simulink model "Frank_mececaneum"  (R2023b)
settings: Solver=VariableStepAuto  StartTime=0.0  StopTime=10.0  RelTol=1e-3
values from neighbouring files (symbols this model uses):
  qn = [0, pi/4, pi, 0, pi/4, 0]    [OMPro.m]    (also in OMPro_v1.m = [0, -pi/4, 0, 0, pi/4, 0]; OManPro.m = rand(1,6); moron9dof.m = [0.1 0.1 pi/4 pi/4 -pi/4 pi/4 0 pi/4 0]; testing2.m = [0 pi/4 pi/4 0 pi/4 0])
undefined symbols (not defined in the file or in its folder): cinertia, nofriction, p560
libraries: roblocks x8
settings Model: Creator=kangwang  LastModifiedBy=kangwang

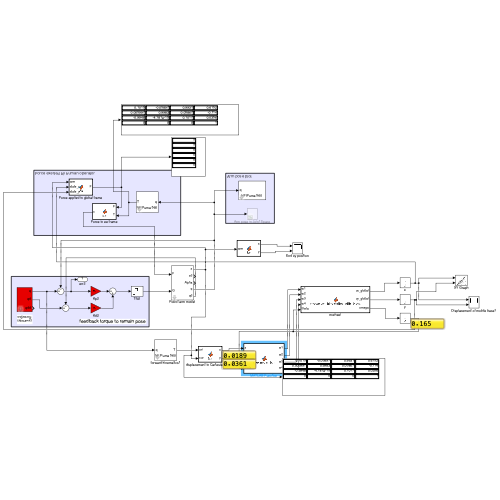
[thumbnail: Simulink's stored preview of the top-level diagram]
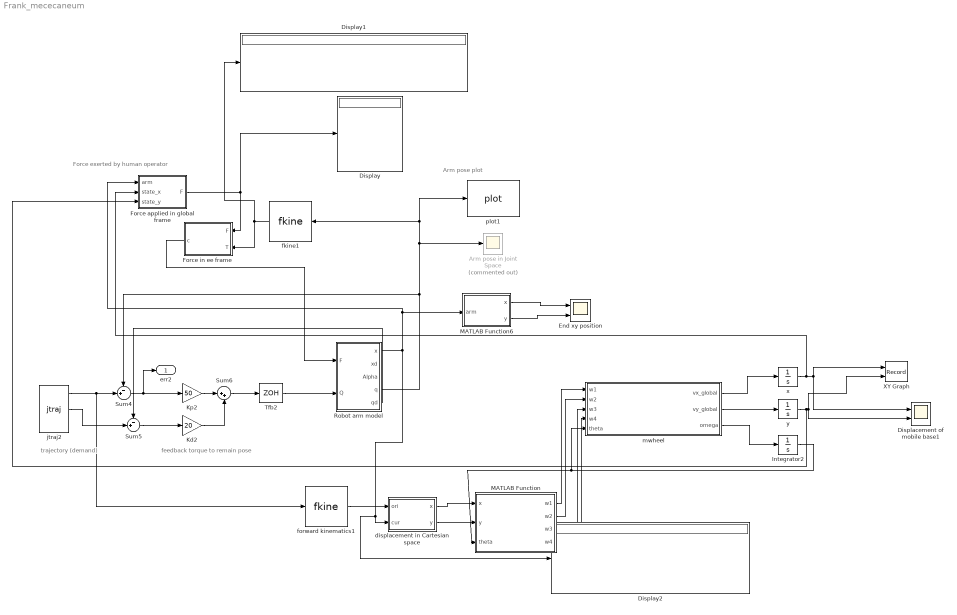
== system Frank_mececaneum ==
  note: feedback torque to remain pose
  note: Force exerted by human operator
  note: trajectory
      | (demand)
  note: Arm pose plot
  Arm pose in Joint Space : Scope  Commented=on
  Displacement of mobile base1 : Scope  NumInputPorts=2
  Display : Display
  Display1 : Display
  Display2 : Display
  End xy position : Scope  NumInputPorts=2
  Force applied in global frame : MATLAB Function  TreatAsAtomicUnit=on
  Force in ee frame : MATLAB Function  TreatAsAtomicUnit=on
  Integrator2 : Integrator
  Kd2 : Gain  Gain=20  SaturateOnIntegerOverflow=on  OutDataTypeStr=Inherit: Same as input  ParamDataTypeStr=Inherit: Same as input
  Kp2 : Gain  Gain=50  SaturateOnIntegerOverflow=on  OutDataTypeStr=Inherit: Same as input  ParamDataTypeStr=Inherit: Same as input
  MATLAB Function : MATLAB Function  TreatAsAtomicUnit=on
  MATLAB Function6 : MATLAB Function  TreatAsAtomicUnit=on
  Robot arm model : Subsystem  mask{robot=nofriction(p560), q0=qn}
      mask prompts: q0 "Initial joint angles"
  Sum4 : Sum  Inputs=-+|  InputSameDT=on  SaturateOnIntegerOverflow=on  OutDataTypeStr=Inherit: Same as first input
  Sum5 : Sum  Inputs=-+|  InputSameDT=on  SaturateOnIntegerOverflow=on  OutDataTypeStr=Inherit: Same as first input
  Sum6 : Sum  Inputs=|++  InputSameDT=on  SaturateOnIntegerOverflow=on  OutDataTypeStr=Inherit: Same as first input
  Tfb2 : ZeroOrderHold  SampleTime=0.002
  XY Graph : Record  FileSettingsInternal="{\"entries\":[{\"content\":{\"excelSettings\":{\"content\":{},\"type\":\"Streamout.ExcelSettings\"}},\"type\":\"Streamout.FileSettingStorage\",\"uuid\":\"\"}],\"packageUris\":[\"http:\\/\\/schema.mathworks.com\\/mf0\\/streamout_blocks\\/R2020a\"],\"version\":\"1.0\"}"  Layout=[1 1]  SignalsInternal="{\"entries\":[{\"content\":{\"signals\":[{\"content\":{\"blockPath\":[],\"dimensions\":[1],\"domain\":\"\",\"lineColor\":\"#a2142f\",\"plots\":[1],\"port\":1,\"sid\":[\"\"],\"signalID\":412,\"signalName\":\"x\"},\"type\":\"RecordBlkView.Signal\",\"uuid\":\"\"},{\"content\":{\"blockPath\":[],\"dimensions\":[1],\"domain\":\"\",\"lineColor\":\"#139fff\",\"plots\":[1],\"port\":2,\"sid\":[\"\"],\"signalID\":416,\"signalName\":\"y\"},\"type\":\"RecordBlkView.Signal\",\"uuid\":\"\"}]},\"type\":\"RecordBlkView.InputSignals\",\"uuid\":\"\"}],\"packageUris\":[\"http:\\/\\/schema.mathworks.com\\/mf0\\/streamout_blocks\\/R2020a\"],\"version\":\"1.0\"}"  VisualizationBindings="{\"xyplotplugin\":{\"info\":[{\"series\":[{\"bindingParametersList\":[{\"parameter\":\"X-Axis\",\"signalID\":412,\"signalName\":\"x\"},{\"parameter\":\"Y-Axis\",\"signalID\":416,\"signalName\":\"y\"}],\"seriesID\":11544}],\"subplotID\":1}]}}"  CompatibilityTag=XY
  displacement in Cartesian space : MATLAB Function  TreatAsAtomicUnit=on
  fkine1 : roblocks/Arm/fkine  robot=nofriction(p560)
  forward kinematics1 : roblocks/Arm/fkine  robot=nofriction(p560)
  jtraj2 : roblocks/Toolbox/jtraj  q0=[0 0.7854 3.1416 0 0.7854 0]  qf=[0 0.7854 3.1416 0 0.7854 0]  tmax=5  ts=0.02
  mwheel : MATLAB Function  TreatAsAtomicUnit=on
  plot1 : roblocks/Arm/plot  robot=nofriction(p560)  fps=10  holdplot=on
  x : Integrator
  y : Integrator
  err2 : Outport
  wires:
  Force in ee frame/1(c) -> Robot arm model/1(F)
  Robot arm model/4(q) -> plot1/1, fkine1/1, Arm pose in Joint Space/1, Sum4/1
  displacement in Cartesian space/1(x) -> MATLAB Function/1(x)
  Sum6/1 -> Tfb2/1
  Robot arm model/1(x) -> MATLAB Function6/1(arm), Force applied in global frame/1(arm), Display2/1, displacement in Cartesian space/2(cur)
  fkine1/1 -> Display1/1, Force in ee frame/2(T)
  Sum5/1 -> Kd2/1
  Robot arm model/5(qd) -> Sum5/1
  Force applied in global frame/1(F) -> Display/1, Force in ee frame/1(F)
  displacement in Cartesian space/2(y) -> MATLAB Function/2(y)
  Tfb2/1 -> Robot arm model/2(Q)
  forward kinematics1/1 -> displacement in Cartesian space/1(ori)
  Kd2/1 -> Sum6/2
  jtraj2/1 -> forward kinematics1/1, Sum4/2
  Kp2/1 -> Sum6/1
  jtraj2/2 -> Sum5/2
  Sum4/1 -> err2/1, Kp2/1
  MATLAB Function6/2(y) -> End xy position/2
  MATLAB Function6/1(x) -> End xy position/1
  mwheel/1(vx_global) -> x/1
  mwheel/2(vy_global) -> y/1
  mwheel/3(omega) -> Integrator2/1
  Integrator2/1 -> MATLAB Function/3(theta), mwheel/5(theta)
  x/1 -> Force applied in global frame/2(state_x), Displacement of mobile base1/1, XY Graph/1
  y/1 -> Force applied in global frame/3(state_y), Displacement of mobile base1/2, XY Graph/2
  MATLAB Function/1(w1) -> mwheel/1(w1)
  MATLAB Function/2(w2) -> mwheel/2(w2)
  MATLAB Function/3(w3) -> mwheel/3(w3)
  MATLAB Function/4(w4) -> mwheel/4(w4)

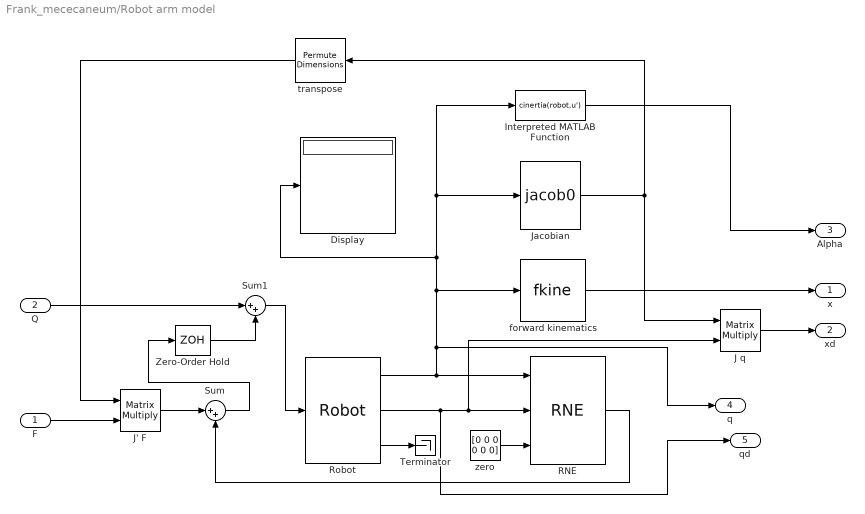
== system Frank_mececaneum/Robot arm model ==
  F : Inport
  Q : Inport  Port=2
  Display : Display
  Interpreted MATLAB Function : MATLABFcn  MATLABFcn=cinertia(robot,u')  OutputDimensions=[6 6]  Output1D=off
  J q : Product  Multiplication=Matrix(*)
  J' F : Product  Multiplication=Matrix(*)
  Jacobian : roblocks/Arm/jacob0   robot=robot
  RNE : roblocks/Arm/RNE  robot=robot  grav=[0 0 9.81]
  Robot : roblocks/Arm/Robot  robot=robot  q0=q0
  Sum : Sum  Inputs=|++
  Sum1 : Sum  Inputs=|++
  Terminator : Terminator
  Zero-Order Hold : ZeroOrderHold  SampleTime=5e-3
  forward kinematics : roblocks/Arm/fkine  robot=robot
  transpose : PermuteDimensions
  zero : Constant  Value=[0 0 0 0 0 0]
  x : Outport
  xd : Outport  Port=2
  Alpha : Outport  Port=3
  q : Outport  Port=4
  qd : Outport  Port=5
  wires:
  Interpreted MATLAB Function/1 -> Alpha/1
  Sum/1 -> Zero-Order Hold/1
  F/1 -> J' F/2
  transpose/1 -> J' F/1
  J' F/1 -> Sum/1
  zero/1 -> RNE/3
  Robot/3 -> Terminator/1
  Robot/2 -> qd/1, RNE/2, J q/2
  Robot/1 -> RNE/1, forward kinematics/1, Interpreted MATLAB Function/1, Jacobian/1, Display/1, q/1
  forward kinematics/1 -> x/1
  J q/1 -> xd/1
  Jacobian/1 -> transpose/1, J q/1
  Q/1 -> Sum1/1
  Sum1/1 -> Robot/1
  Zero-Order Hold/1 -> Sum1/2
  RNE/1 -> Sum/2

== matlab function Frank_mececaneum/MATLAB Function ==
  data: x input; w1 output; y input; theta input; w2 output; w3 output; w4 output
function [w1, w2, w3, w4] = mecanum_fcn(x, y, theta)

    % Robot parameters
    r = 0.05;  % wheel radius [m]
    L = 0.3;   % robot length
    W = 0.2;   % robot width

    % --- Step 1: Scaling and direction ---
    y_scale = 0.522;
    x_scale = 1.0;

    x_scaled = x_scale * x;
    y_scaled = y_scale * y;

    % Step 2: Desired direction of motion
    force_angle = atan2(y_scaled, x_scaled);

    % Step 3: Compute forward and lateral velocities in robot frame
    speed = 0.5 * norm([x_scaled, y_scaled]); % adjust gain as needed
    error_theta = wrapToPi(force_angle - theta);

    % Rotation speed to align robot
    k_theta = 2.0;
    omega = k_theta * error_theta;

    % Desired direction in global frame
    vx_global = speed * cos(force_angle);
    vy_global = speed * sin(force_angle);

    % Convert to robot frame (inverse rotation)
    vx = cos(theta) * vx_global + sin(theta) * vy_global;
    vy = -sin(theta) * vx_global + cos(theta) * vy_global;

    % --- Step 4: Inverse kinematics to compute wheel speeds ---
    M = (1/r) * [
        1, -1, -(L + W);   % Front Left
        1,  1,  (L + W);   % Front Right
        1,  1, -(L + W);   % Rear Left
        1, -1,  (L + W)    % Rear Right
    ];

    v = [vx; vy; omega];
    w = M * v;

    % Assign outputs
    w1 = w(1);
    w2 = w(2);
    w3 = w(3);
    w4 = w(4);
end

== matlab function Frank_mececaneum/mwheel ==
  data: w1 input; vx_global output; w2 input; w3 input; w4 input; vy_global output; omega output; theta input
function [vx_global, vy_global, omega] = mecanum_kinematics_with_theta(w1, w2, w3, w4, theta)
    % Robot physical parameters
    r = 0.05;   % wheel radius [m]
    L = 0.3;    % robot length [m]
    W = 0.2;    % robot width [m]

    % Compute local frame velocities
    vx = r/4 * (w1 + w2 + w3 + w4);
    vy = r/4 * (-w1 + w2 - w3 + w4);
    omega = r/(4*(L + W)) * (-w1 + w2 + w3 - w4);

    % Rotate to global frame using current theta
    vx_global = vx * cos(theta) - vy * sin(theta);
    vy_global = vx * sin(theta) + vy * cos(theta);
end

== matlab function Frank_mececaneum/Force in ee frame ==
  data: F input; T input; c output
function c = fcn(F, T)
F(1:3)
inv(T(1:3,1:3))
y = inv(T(1:3,1:3))*F(1:3);
c = [y.', 0,0,0].'

== matlab function Frank_mececaneum/displacement in Cartesian space ==
  data: x output; ori input; y output; cur input
function [x,y]= fcn(ori, cur)
x = cur(1,4)-ori(1,4);
y = cur(2,4)-ori(2,4);

== matlab function Frank_mececaneum/Force applied in global frame ==
  data: arm input; F output; state_x input; state_y input
function F = fcn(arm,state_x,state_y)
x_arm = arm(1,4);
x_base = state_x;
y_arm = arm(2,4);
y_base = state_y;
x = x_base+x_arm;
y = y_base+y_arm;
F = [0 0 0 0 0 0].';
if x < 1.2 || y < 1.8 
    F = [5 5 0 0 0 0].';
end

== matlab function Frank_mececaneum/MATLAB Function6 ==
  data: x output; arm input; y output
function [x,y]= fcn(arm)
x = arm(1,4);
y = arm(2,4);
